simulink model "PIDControl3Axis"  (R2024b)
settings: Solver=ode45  StartTime=0.0  StopTime=20  RelTol=1e-3
settings Model: Creator=mkozl  LastModifiedBy=mkozl

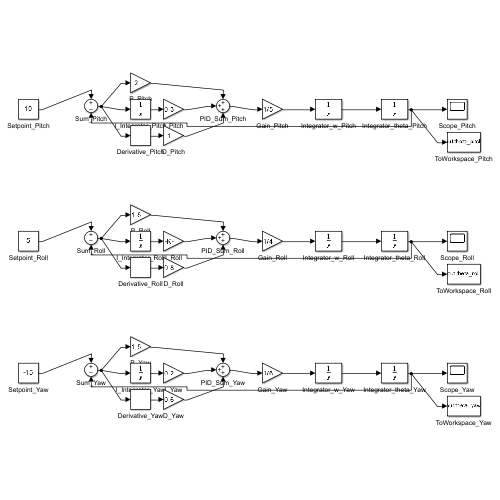
[thumbnail: Simulink's stored preview of the top-level diagram]
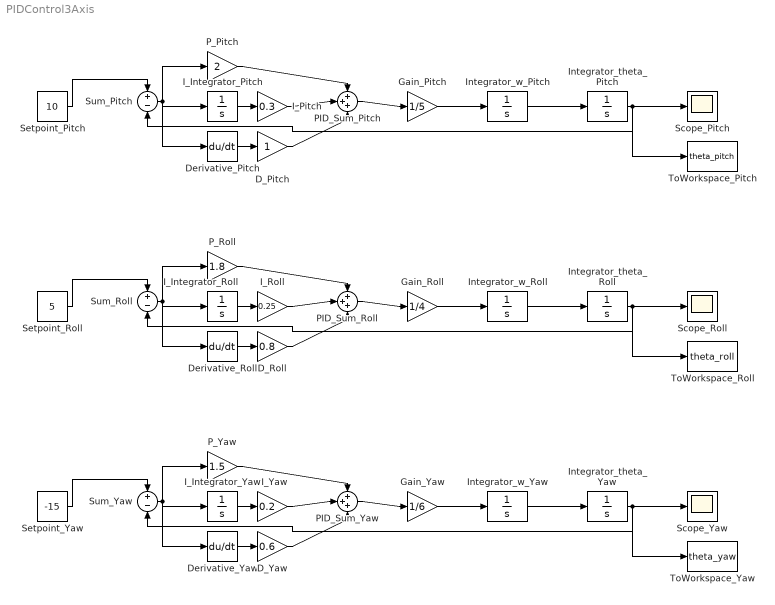
== system PIDControl3Axis ==
  D_Pitch : Gain
  D_Roll : Gain  Gain=0.8
  D_Yaw : Gain  Gain=0.6
  Derivative_Pitch : Derivative
  Derivative_Roll : Derivative
  Derivative_Yaw : Derivative
  Gain_Pitch : Gain  Gain=1/5
  Gain_Roll : Gain  Gain=1/4
  Gain_Yaw : Gain  Gain=1/6
  I_Integrator_Pitch : Integrator
  I_Integrator_Roll : Integrator
  I_Integrator_Yaw : Integrator
  I_Pitch : Gain  Gain=0.3
  I_Roll : Gain  Gain=0.25
  I_Yaw : Gain  Gain=0.2
  Integrator_theta_Pitch : Integrator
  Integrator_theta_Roll : Integrator
  Integrator_theta_Yaw : Integrator
  Integrator_w_Pitch : Integrator
  Integrator_w_Roll : Integrator
  Integrator_w_Yaw : Integrator
  PID_Sum_Pitch : Sum  Inputs=+++
  PID_Sum_Roll : Sum  Inputs=+++
  PID_Sum_Yaw : Sum  Inputs=+++
  P_Pitch : Gain  Gain=2
  P_Roll : Gain  Gain=1.8
  P_Yaw : Gain  Gain=1.5
  Scope_Pitch : Scope
  Scope_Roll : Scope
  Scope_Yaw : Scope
  Setpoint_Pitch : Constant  Value=10
  Setpoint_Roll : Constant  Value=5
  Setpoint_Yaw : Constant  Value=-15
  Sum_Pitch : Sum  Inputs=+-
  Sum_Roll : Sum  Inputs=+-
  Sum_Yaw : Sum  Inputs=+-
  ToWorkspace_Pitch : ToWorkspace  VariableName=theta_pitch  SaveFormat=Structure With Time  SampleTime=-1
  ToWorkspace_Roll : ToWorkspace  VariableName=theta_roll  SaveFormat=Structure With Time  SampleTime=-1
  ToWorkspace_Yaw : ToWorkspace  VariableName=theta_yaw  SaveFormat=Structure With Time  SampleTime=-1
  wires:
  Setpoint_Pitch/1 -> Sum_Pitch/1
  Sum_Pitch/1 -> P_Pitch/1, I_Integrator_Pitch/1, Derivative_Pitch/1
  P_Pitch/1 -> PID_Sum_Pitch/1
  I_Integrator_Pitch/1 -> I_Pitch/1
  I_Pitch/1 -> PID_Sum_Pitch/2
  Derivative_Pitch/1 -> D_Pitch/1
  D_Pitch/1 -> PID_Sum_Pitch/3
  PID_Sum_Pitch/1 -> Gain_Pitch/1
  Gain_Pitch/1 -> Integrator_w_Pitch/1
  Integrator_w_Pitch/1 -> Integrator_theta_Pitch/1
  Integrator_theta_Pitch/1 -> Scope_Pitch/1, ToWorkspace_Pitch/1, Sum_Pitch/2
  Setpoint_Roll/1 -> Sum_Roll/1
  Sum_Roll/1 -> P_Roll/1, I_Integrator_Roll/1, Derivative_Roll/1
  P_Roll/1 -> PID_Sum_Roll/1
  I_Integrator_Roll/1 -> I_Roll/1
  I_Roll/1 -> PID_Sum_Roll/2
  Derivative_Roll/1 -> D_Roll/1
  D_Roll/1 -> PID_Sum_Roll/3
  PID_Sum_Roll/1 -> Gain_Roll/1
  Gain_Roll/1 -> Integrator_w_Roll/1
  Integrator_w_Roll/1 -> Integrator_theta_Roll/1
  Integrator_theta_Roll/1 -> Scope_Roll/1, ToWorkspace_Roll/1, Sum_Roll/2
  Setpoint_Yaw/1 -> Sum_Yaw/1
  Sum_Yaw/1 -> P_Yaw/1, I_Integrator_Yaw/1, Derivative_Yaw/1
  P_Yaw/1 -> PID_Sum_Yaw/1
  I_Integrator_Yaw/1 -> I_Yaw/1
  I_Yaw/1 -> PID_Sum_Yaw/2
  Derivative_Yaw/1 -> D_Yaw/1
  D_Yaw/1 -> PID_Sum_Yaw/3
  PID_Sum_Yaw/1 -> Gain_Yaw/1
  Gain_Yaw/1 -> Integrator_w_Yaw/1
  Integrator_w_Yaw/1 -> Integrator_theta_Yaw/1
  Integrator_theta_Yaw/1 -> Scope_Yaw/1, ToWorkspace_Yaw/1, Sum_Yaw/2
